simulink model "ortho_CAN_controlV2"  (R2016b)
settings: Solver=FixedStepDiscrete  StartTime=0.0  StopTime=180  FixedStep=.001  RelTol=1e-3  EnableMultiTasking=on
values from neighbouring files (symbols this model uses):
  rho1 = (rho01*(1-d(3)))+(rho11*d(3))    [fcn.m]
  rho2 = (rho02*(1-d(3)))+(rho12*d(3))    [fcn.m]
  theta1 = (theta01*(1-d(3)))+(theta11*d(3))    [fcn.m]
  theta2 = (theta02*(1-d(3)))+(theta12*d(3))    [fcn.m]
undefined symbols (not defined in the file or in its folder): bit, fdesignblkfcn, gcbh, rho_end, Standard, theta_end
libraries: slrtlib x7, simulink x6, slrtsoftinglib x3, xpcnilib x3, canmsglib x2
(part 1 of 2)
settings Model: xpc_rtwmakecfg_data=_xpccanac2pci_  SimulationMode=external  Creator=dholley  LastModifiedBy=1108gotthem
settings SolverCC: EnableConcurrentExecution=on  AlgebraicLoopSolver=LineSearch
settings DataIOCC: LimitDataPoints=on  SaveFormat=Array  SaveOutput=off  SignalLogging=off  DSMLogging=off
settings OptimizationCC: BlockReduction=off  OptimizeBlockIOStorage=off  BufferReuse=off  GlobalBufferReuse=off  ExpressionFolding=off  LocalBlockOutputs=off
settings DebuggingCC: UnderspecifiedInitializationDetection=Classic  MergeDetectMultiDrivingBlocksExec=none  SolverPrmCheckMsg=warning  StateNameClashWarn=warning  SFUnexpectedBacktrackingDiag=warning  SFNoUnconditionalDefaultTransitionDiag=warning  SFExecutionAtInitializationDiag=none
settings HardwareCC: ProdBitPerPointer=32  ProdBitPerSizeT=32  ProdBitPerPtrDiffT=32  ProdLargestAtomicFloat=None  ProdWordSize=32  ProdLongLongMode=on  ProdHWDeviceType=Generic->32-bit x86 compatible
settings ModelReferenceCC: PropagateSignalLabelsOutOfModel=off
settings RTWCC: SystemTargetFile=slrt.tlc  TemplateMakefile=slrt_default_tmf  Description=Simulink Real-Time  RTWCompilerOptimization=on
settings SimulinkRealTimeCC: RL32LogBufSizeModifier=6120000  xPCisModelTimeout=off  xPCModelTimeoutSecs=120
settings ConfigComp: CovMetricSettings=dw  CovHtmlReporting=on  CovSaveCumulativeToWorkspaceVar=on  CovSaveSingleToWorkspaceVar=on  CovExternalEMLEnable=off

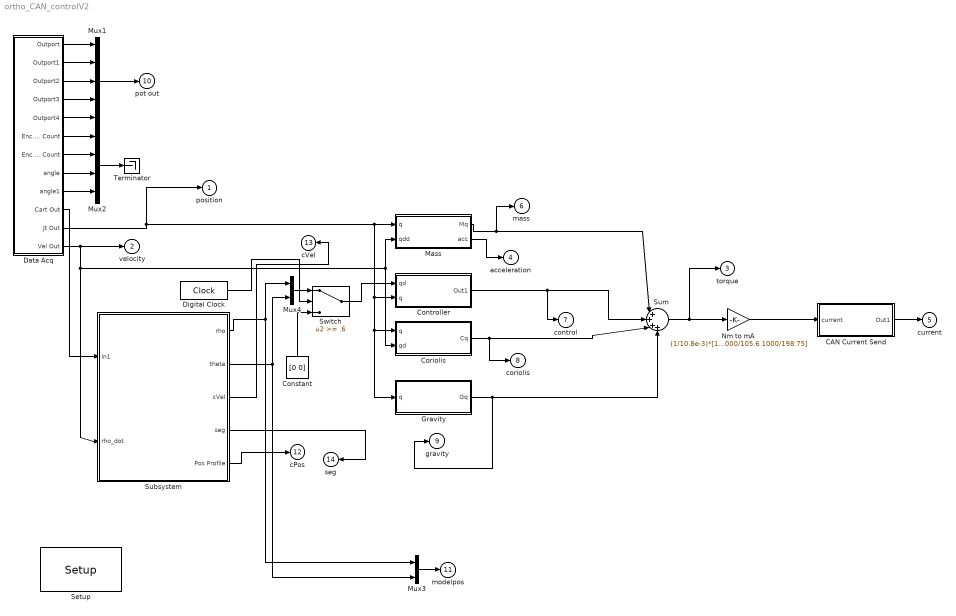
== system ortho_CAN_controlV2 ==
  CAN Current Send : Subsystem
  Constant : Constant  Value=[0 0]
  Controller : Subsystem  TreatAsAtomicUnit=on
      settings: RTWSystemCode=Inline
  Coriolis : Subsystem  TreatAsAtomicUnit=on
      settings: RTWSystemCode=Inline
  Data Acq : Subsystem
  Digital Clock : DigitalClock  SampleTime=.001
  Gravity : Subsystem  TreatAsAtomicUnit=on
      settings: RTWSystemCode=Inline
  Mass : Subsystem  TreatAsAtomicUnit=on
      settings: RTWSystemCode=Inline
  Mux1 : Mux  Inputs=5
  Mux2 : Mux
  Mux3 : Mux  Inputs=2
  Mux4 : Mux  Inputs=2
  Nm to mA : Gain  Gain=(1/10.8e-3)*[1000/105.6 1000/198.75]
  "Setup " : slrtsoftinglib/CAN-AC2-PCI SJA 1000/Setup   board=1  can1bus=Highspeed (ISO 11898)  can1Baudrate=1 MBaud  can1UserBR=[1,1,4,3]  can2bus=Highspeed (ISO 11898)  can2Baudrate=1 MBaud  can2UserBR=[1,1,4,3]  init=pdo_start  term=pdo_stop  bus_off_out=off  bus_off_rec=Off  ioBaseAddress=-1
  Subsystem : Subsystem
  Sum : Sum  Inputs=|++++
  Switch : Switch  Threshold=.6  SampleTime=.001
  Terminator : Terminator
  position : Outport  InitialOutput=0
  velocity : Outport  Port=2  InitialOutput=0
  torque : Outport  Port=3  InitialOutput=0
  acceleration : Outport  Port=4  InitialOutput=0
  current : Outport  Port=5  InitialOutput=0
  mass : Outport  Port=6  InitialOutput=0
  control : Outport  Port=7  InitialOutput=0
  coriolis : Outport  Port=8  InitialOutput=0
  gravity : Outport  Port=9  InitialOutput=0
  "pot out " : Outport  Port=10  InitialOutput=0
  "modelpos " : Outport  Port=11  InitialOutput=0
  cPos : Outport  Port=12  InitialOutput=0
  cVel : Outport  Port=13  InitialOutput=0
  "seg " : Outport  Port=14  InitialOutput=0
  wires:
  Gravity/1(Gq) -> Sum/4, gravity/1
  Coriolis/1(Cq) -> coriolis/1, Sum/3
  Mass/1(Mq) -> Sum/1, mass/1
  Mass/2(acc) -> acceleration/1
  CAN Current Send/1(Out1) -> current/1
  Data Acq/12(Vel Out) -> velocity/1, Subsystem/2(rho_dot), Coriolis/2(qd), Mass/2(qdd)
  Data Acq/11(Jt Out) -> position/1, Gravity/1(q), Coriolis/1(q), Controller/2(q), Mass/1(q)
  Data Acq/1(Outport) -> Mux1/1
  Data Acq/2(Outport1) -> Mux1/2
  Data Acq/3(Outport2) -> Mux1/3
  Data Acq/4(Outport3) -> Mux1/4
  Data Acq/5(Outport4) -> Mux1/5
  Mux1/1 -> "pot out "/1
  Data Acq/6(Enc. 1 Count) -> Mux2/1
  Data Acq/8(angle) -> Mux2/3
  Mux2/1 -> Terminator/1
  Controller/1(Out1) -> control/1, Sum/2
  Subsystem/1(rho) -> Mux4/1, Mux3/1
  Subsystem/2("theta ") -> Mux4/2, Mux3/2
  Mux3/1 -> "modelpos "/1
  Nm to mA/1 -> CAN Current Send/1(current)
  Sum/1 -> torque/1, Nm to mA/1
  Subsystem/3("cVel ") -> cVel/1
  Subsystem/4("seg ") -> "seg "/1
  Data Acq/7(Enc. 2 Count) -> Mux2/2
  Data Acq/9(angle1) -> Mux2/4
  Data Acq/10(Cart Out) -> Subsystem/1(In1)
  Subsystem/5(Pos Profile) -> cPos/1
  Mux4/1 -> Switch/1
  Switch/1 -> Controller/1(qd)
  Constant/1 -> Switch/3
  Digital Clock/1 -> Switch/2

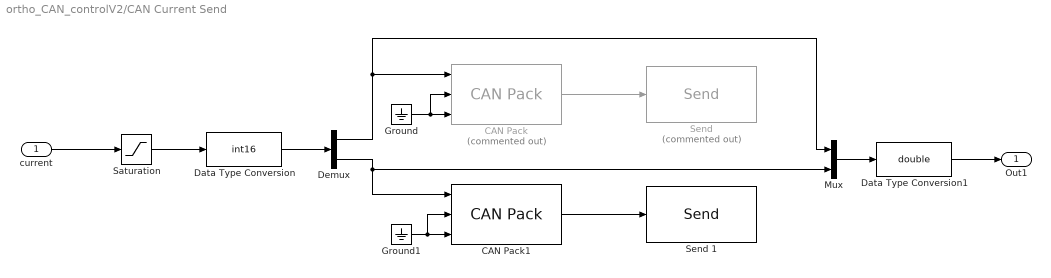
== system ortho_CAN_controlV2/CAN Current Send ==
  current : Inport
  CAN Pack : canmsglib/CAN Pack  Commented=on  MsgList=(none)  MsgName=CAN Msg  MsgIDType=Standard (11-bit identifier)  MsgIdentifier=hex2dec('202')  MsgLength=8  SignalInfo=current$0$16$1$1$1$0$1$0$-Inf$Inf$#null$16$32$1$1$1$0$1$0$-Inf$Inf$#null2$48$16$1$1$1$0$1$0$-Inf$Inf$#  NSignals=3  StartBits=str2num('[int32(0);int32(16);int32(48)]')  SignalSizes=str2num('[int32(16);int32(32);int32(16)]')  ByteOrders=str2num('[int32(1);int32(1);int32(1)]')  DataTypes=str2num('[int32(1);int32(1);int32(1)]')  MultiplexTypes=str2num('[int32(1);int32(1);int32(1)]')  MultiplexValues=str2num('[double(0);double(0);double(0)]')  Factors=str2num('[double(1);double(1);double(1)]')  Offsets=str2num('[double(0);double(0);double(0)]')  Minimums=str2num('[double(-Inf);double(-Inf);double(-Inf)]')  Maximums=str2num('[double(Inf);double(Inf);double(Inf)]')  Remote=off
      settings: DataFormat=manually specified signals
  CAN Pack1 : canmsglib/CAN Pack  MsgList=(none)  MsgName=CAN Msg  MsgIDType=Standard (11-bit identifier)  MsgIdentifier=hex2dec('201')  MsgLength=8  SignalInfo=current$0$16$1$1$1$0$1$0$-Inf$Inf$#null$16$32$1$1$1$0$1$0$-Inf$Inf$#null2$48$16$1$1$1$0$1$0$-Inf$Inf$#  NSignals=3  StartBits=str2num('[int32(0);int32(16);int32(48)]')  SignalSizes=str2num('[int32(16);int32(32);int32(16)]')  ByteOrders=str2num('[int32(1);int32(1);int32(1)]')  DataTypes=str2num('[int32(1);int32(1);int32(1)]')  MultiplexTypes=str2num('[int32(1);int32(1);int32(1)]')  MultiplexValues=str2num('[double(0);double(0);double(0)]')  Factors=str2num('[double(1);double(1);double(1)]')  Offsets=str2num('[double(0);double(0);double(0)]')  Minimums=str2num('[double(-Inf);double(-Inf);double(-Inf)]')  Maximums=str2num('[double(Inf);double(Inf);double(Inf)]')  Remote=off
      settings: DataFormat=manually specified signals
  Data Type Conversion : DataTypeConversion  OutDataTypeStr=int16
  Data Type Conversion1 : DataTypeConversion  OutDataTypeStr=double
  Demux : Demux  Outputs=2
  Ground : Ground
  Ground1 : Ground
  Mux : Mux  Inputs=2
  Saturation : Saturate  UpperLimit=1700  LowerLimit=-1700
  "Send " : slrtsoftinglib/CAN-AC2-PCI SJA 1000/Send   Commented=on  board=1  canPort=CAN 1  range=Standard (11-bit)  ids=hex2dec('202')  sizes=[8]  output=off  ts=0.001  ididx=[2]
  Send 1 : slrtsoftinglib/CAN-AC2-PCI SJA 1000/Send   board=1  canPort=CAN 1  range=Standard (11-bit)  ids=hex2dec('201')  sizes=[8]  output=off  ts=0.001  ididx=[1]
  Out1 : Outport
  wires:
  current/1 -> Saturation/1
  CAN Pack/1 -> "Send "/1
  CAN Pack1/1 -> Send 1/1
  Ground/1 -> CAN Pack/2, CAN Pack/3
  Ground1/1 -> CAN Pack1/2, CAN Pack1/3
  Demux/1 -> CAN Pack/1, Mux/1
  Demux/2 -> Mux/2, CAN Pack1/1
  Saturation/1 -> Data Type Conversion/1
  Data Type Conversion/1 -> Demux/1
  Data Type Conversion1/1 -> Out1/1
  Mux/1 -> Data Type Conversion1/1

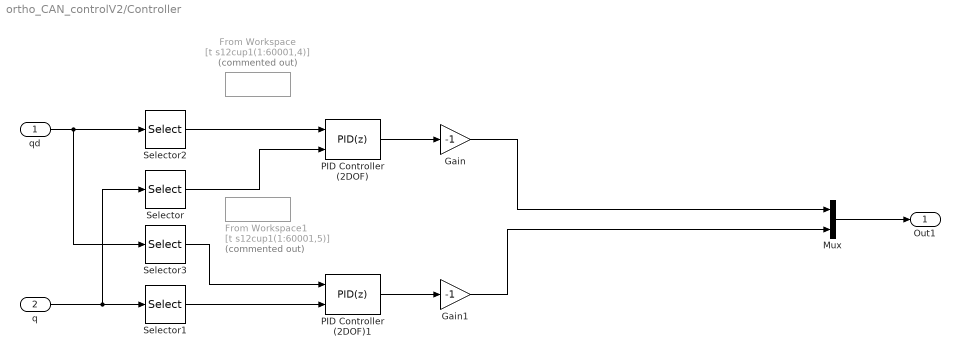
== system ortho_CAN_controlV2/Controller ==
  qd : Inport
  q : Inport  Port=2
  From Workspace : FromWorkspace  Commented=on  VariableName=[t s12cup1(1:60001,4)]  SampleTime=0
  From Workspace1 : FromWorkspace  Commented=on  VariableName=[t s12cup1(1:60001,5)]  SampleTime=0
  Gain : Gain  Gain=-1
  Gain1 : Gain  Gain=-1
  Mux : Mux  Inputs=2
  PID Controller (2DOF) : simulink/Continuous/PID Controller (2DOF)  Controller=PID  TimeDomain=Discrete-time  SampleTime=.001  IntegratorMethod=Forward Euler  FilterMethod=Forward Euler  Form=Parallel  UseFilter=on  ControllerParametersSource=internal  P=75  I=45  D=2  N=103  b=1  c=1  InitialConditionSource=internal  InitialConditionForIntegrator=0  InitialConditionForFilter=0  ExternalReset=none  LimitOutput=off  UpperSaturationLimit=inf  LowerSaturationLimit=-inf  LinearizeAsGain=on  AntiWindupMode=none  Kb=1  TrackingMode=off  Kt=1  PParamMin=[]  PParamMax=[]  IParamMin=[]  IParamMax=[]  DParamMin=[]  DParamMax=[]  NParamMin=[]  NParamMax=[]  bParamMin=[]  bParamMax=[]  cParamMin=[]  cParamMax=[]  KbParamMin=[]  KbParamMax=[]  KtParamMin=[]  KtParamMax=[]  POutMin=[]  POutMax=[]  IOutMin=[]  IOutMax=[]  DOutMin=[]  DOutMax=[]  NOutMin=[]  NOutMax=[]  bOutMin=[]  bOutMax=[]  cOutMin=[]  cOutMax=[]  KbOutMin=[]  KbOutMax=[]  KtOutMin=[]  KtOutMax=[]  IntegratorOutMin=[]  IntegratorOutMax=[]  FilterOutMin=[]  FilterOutMax=[]  SumOutMin=[]  SumOutMax=[]  Sum1OutMin=[]  Sum1OutMax=[]  Sum2OutMin=[]  Sum2OutMax=[]  Sum3OutMin=[]  Sum3OutMax=[]  SumI1OutMin=[]  SumI1OutMax=[]  SumI2OutMin=[]  SumI2OutMax=[]  SumI3OutMin=[]  SumI3OutMax=[]  SumDOutMin=[]  SumDOutMax=[]  SaturationOutMin=[]  SaturationOutMax=[]  IntegratorContinuousStateAttributes=''  IntegratorStateMustResolveToSignalObject=off  IntegratorRTWStateStorageClass=Auto  FilterContinuousStateAttributes=''  FilterStateMustResolveToSignalObject=off  FilterRTWStateStorageClass=Auto  DifferentiatorICPrevScaledInput=0  DifferentiatorOutMin=[]  DifferentiatorOutMax=[]
  PID Controller (2DOF)1 : simulink/Continuous/PID Controller (2DOF)  Controller=PID  TimeDomain=Discrete-time  SampleTime=.001  IntegratorMethod=Forward Euler  FilterMethod=Forward Euler  Form=Parallel  UseFilter=on  ControllerParametersSource=internal  P=30  I=20  D=3  N=100  b=1  c=1  InitialConditionSource=internal  InitialConditionForIntegrator=0  InitialConditionForFilter=0  ExternalReset=none  LimitOutput=off  UpperSaturationLimit=inf  LowerSaturationLimit=-inf  LinearizeAsGain=on  AntiWindupMode=none  Kb=1  TrackingMode=off  Kt=1  PParamMin=[]  PParamMax=[]  IParamMin=[]  IParamMax=[]  DParamMin=[]  DParamMax=[]  NParamMin=[]  NParamMax=[]  bParamMin=[]  bParamMax=[]  cParamMin=[]  cParamMax=[]  KbParamMin=[]  KbParamMax=[]  KtParamMin=[]  KtParamMax=[]  POutMin=[]  POutMax=[]  IOutMin=[]  IOutMax=[]  DOutMin=[]  DOutMax=[]  NOutMin=[]  NOutMax=[]  bOutMin=[]  bOutMax=[]  cOutMin=[]  cOutMax=[]  KbOutMin=[]  KbOutMax=[]  KtOutMin=[]  KtOutMax=[]  IntegratorOutMin=[]  IntegratorOutMax=[]  FilterOutMin=[]  FilterOutMax=[]  SumOutMin=[]  SumOutMax=[]  Sum1OutMin=[]  Sum1OutMax=[]  Sum2OutMin=[]  Sum2OutMax=[]  Sum3OutMin=[]  Sum3OutMax=[]  SumI1OutMin=[]  SumI1OutMax=[]  SumI2OutMin=[]  SumI2OutMax=[]  SumI3OutMin=[]  SumI3OutMax=[]  SumDOutMin=[]  SumDOutMax=[]  SaturationOutMin=[]  SaturationOutMax=[]  IntegratorContinuousStateAttributes=''  IntegratorStateMustResolveToSignalObject=off  IntegratorRTWStateStorageClass=Auto  FilterContinuousStateAttributes=''  FilterStateMustResolveToSignalObject=off  FilterRTWStateStorageClass=Auto  DifferentiatorICPrevScaledInput=0  DifferentiatorOutMin=[]  DifferentiatorOutMax=[]
  Selector : Selector  InputPortWidth=2  IndexOptions=Index vector (dialog)  Indices=[1]  OutputSizes=1
  Selector1 : Selector  InputPortWidth=2  IndexOptions=Index vector (dialog)  Indices=[2]  OutputSizes=1
  Selector2 : Selector  InputPortWidth=2  IndexOptions=Index vector (dialog)  Indices=[1]  OutputSizes=1
  Selector3 : Selector  InputPortWidth=2  IndexOptions=Index vector (dialog)  Indices=[2]  OutputSizes=1
  Out1 : Outport
  wires:
  q/1 -> Selector/1, Selector1/1
  Selector/1 -> PID Controller (2DOF)/2
  Mux/1 -> Out1/1
  Selector1/1 -> PID Controller (2DOF)1/2
  PID Controller (2DOF)/1 -> Gain/1
  PID Controller (2DOF)1/1 -> Gain1/1
  Gain/1 -> Mux/1
  Gain1/1 -> Mux/2
  qd/1 -> Selector3/1, Selector2/1
  Selector2/1 -> PID Controller (2DOF)/1
  Selector3/1 -> PID Controller (2DOF)1/1

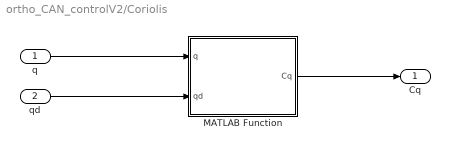
== system ortho_CAN_controlV2/Coriolis ==
  q : Inport
  qd : Inport  Port=2
  MATLAB Function : MATLAB Function  TreatAsAtomicUnit=on
  Cq : Outport
  wires:
  q/1 -> MATLAB Function/1(q)
  MATLAB Function/1(Cq) -> Cq/1
  qd/1 -> MATLAB Function/2(qd)

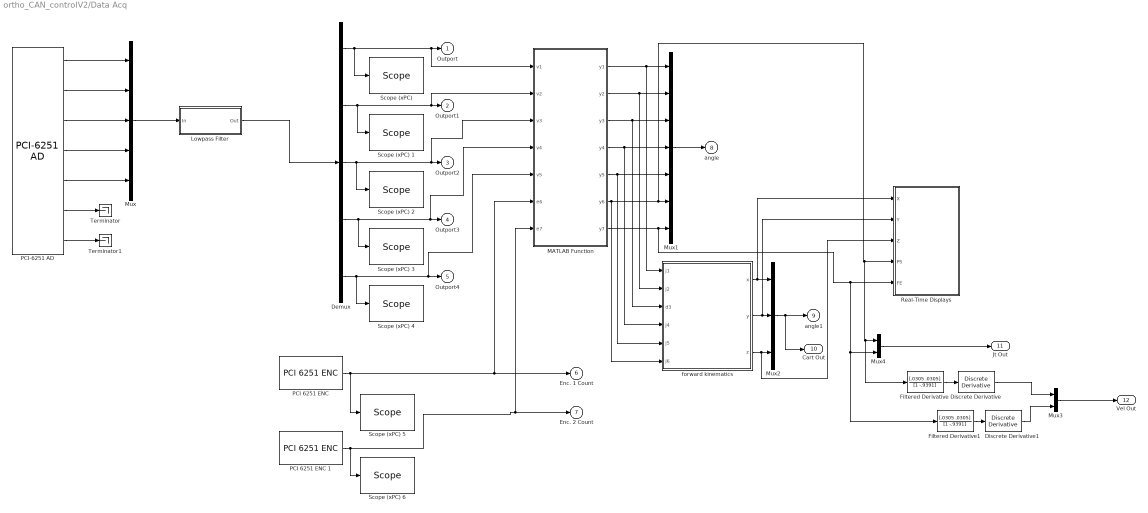
== system ortho_CAN_controlV2/Data Acq ==
  Demux : Demux  Outputs=5
  Discrete Derivative : simulink/Discrete/Discrete Derivative  gainval=1.0  ICPrevScaledInput=0.0  OutMin=[]  OutMax=[]  OutDataType=fixdt(1, 16)  OutScaling=2^-10  DoSatur=off
  Discrete Derivative1 : simulink/Discrete/Discrete Derivative  gainval=1.0  ICPrevScaledInput=0.0  OutMin=[]  OutMax=[]  OutDataType=fixdt(1, 16)  OutScaling=2^-10  DoSatur=off
  Filtered Derivative : DiscreteFilter  Numerator=[.0305 .0305]  Denominator=[1 -.9391]  SampleTime=0.001
  Filtered Derivative1 : DiscreteFilter  Numerator=[.0305 .0305]  Denominator=[1 -.9391]  SampleTime=0.001
  Lowpass Filter : Subsystem  DialogController=fdesignblkfcn  InitFcn=fdesignblkfcn(gcbh, {'InitFcn'});  mask(Lowpass Filter){}
      mask help: Design a lowpass filter
      settings: CopyFcn=fdesignblkfcn(gcbh, {'CopyFcn'});
      mask Help: helpview(mapfilelocation('dsp'), 'dsplowpassfilter');
      mask Display: disp('Lowpass')
  MATLAB Function : MATLAB Function  TreatAsAtomicUnit=on
  Mux : Mux  Inputs=5
  Mux1 : Mux  Inputs=7
  Mux2 : Mux  Inputs=3
  Mux3 : Mux  Inputs=2
  Mux4 : Mux  Inputs=2
  "PCI 6251 ENC " : xpcnilib/Incremental Encoder/PCI 6251 ENC   channel=1  countMode=Quadrature Mode x4  initCount=0  reload=off  indexPhase=A low B low  filter=None  sampleTime=0.001  slot=-1
  PCI 6251 ENC 1 : xpcnilib/Incremental Encoder/PCI 6251 ENC   channel=0  countMode=Quadrature Mode x4  initCount=0  reload=off  indexPhase=A low B low  filter=None  sampleTime=0.001  slot=-1
  PCI-6251 AD : xpcnilib/A//D/M Series/PCI-6251 AD  channel=[1,2,3,4,5,7,8]  range=[10,10,10,10,10,10,10]  coupling=[1,1,1,1,1,2,2]  scantime=5e-6  sampletime=0.001  slot=-1
  "Real-Time Displays " : Subsystem
  "Scope (xPC) " : slrtlib/Displays and Logging/Scope   scopeno=5  scopetype=Target  autostart=on  viewmode=Graphical rolling  formatstr='%15.6f'  grid=on  ylimits=[0,10]  nosamples=15001  noprepostsamples=0  interleave=1  triggermode=FreeRun  triggersignal=1  trigsignalfromport=off  triggerlevel=0.0  triggerslope=Either  triggerscope=1  triggersample=0  filename=data.dat  mode=Lazy  writesize=512  autorestart=off  dynamicfilemode=off  maxwritefilesize=512*1024^2
  Scope (xPC) 1 : slrtlib/Displays and Logging/Scope   scopeno=6  scopetype=Target  autostart=on  viewmode=Graphical rolling  formatstr='%15.6f'  grid=on  ylimits=[0,10]  nosamples=15001  noprepostsamples=0  interleave=1  triggermode=FreeRun  triggersignal=1  trigsignalfromport=off  triggerlevel=0.0  triggerslope=Either  triggerscope=1  triggersample=0  filename=data.dat  mode=Lazy  writesize=512  autorestart=off  dynamicfilemode=off  maxwritefilesize=512*1024^2
  Scope (xPC) 2 : slrtlib/Displays and Logging/Scope   scopeno=1  scopetype=Target  autostart=on  viewmode=Graphical rolling  formatstr='%15.6f'  grid=on  ylimits=[0,10]  nosamples=15001  noprepostsamples=0  interleave=1  triggermode=FreeRun  triggersignal=1  trigsignalfromport=off  triggerlevel=0.0  triggerslope=Either  triggerscope=1  triggersample=0  filename=data.dat  mode=Lazy  writesize=512  autorestart=off  dynamicfilemode=off  maxwritefilesize=512*1024^2
  Scope (xPC) 3 : slrtlib/Displays and Logging/Scope   scopeno=2  scopetype=Target  autostart=on  viewmode=Graphical rolling  formatstr='%15.6f'  grid=on  ylimits=[0,10]  nosamples=15001  noprepostsamples=0  interleave=1  triggermode=FreeRun  triggersignal=1  trigsignalfromport=off  triggerlevel=0.0  triggerslope=Either  triggerscope=1  triggersample=0  filename=data.dat  mode=Lazy  writesize=512  autorestart=off  dynamicfilemode=off  maxwritefilesize=512*1024^2
  Scope (xPC) 4 : slrtlib/Displays and Logging/Scope   scopeno=3  scopetype=Target  autostart=on  viewmode=Graphical rolling  formatstr='%15.6f'  grid=on  ylimits=[0,10]  nosamples=15001  noprepostsamples=0  interleave=1  triggermode=FreeRun  triggersignal=1  trigsignalfromport=off  triggerlevel=0.0  triggerslope=Either  triggerscope=1  triggersample=0  filename=data.dat  mode=Lazy  writesize=512  autorestart=off  dynamicfilemode=off  maxwritefilesize=512*1024^2
  Scope (xPC) 5 : slrtlib/Displays and Logging/Scope   scopeno=7  scopetype=Target  autostart=on  viewmode=Graphical rolling  formatstr='%15.6f'  grid=on  ylimits=[-15000,15000]  nosamples=15001  noprepostsamples=0  interleave=1  triggermode=FreeRun  triggersignal=1  trigsignalfromport=off  triggerlevel=0.0  triggerslope=Either  triggerscope=1  triggersample=0  filename=data.dat  mode=Lazy  writesize=512  autorestart=off  dynamicfilemode=off  maxwritefilesize=512*1024^2
  Scope (xPC) 6 : slrtlib/Displays and Logging/Scope   scopeno=4  scopetype=Target  autostart=on  viewmode=Graphical rolling  formatstr='%15.6f'  grid=on  ylimits=[-40000,40000]  nosamples=15001  noprepostsamples=0  interleave=1  triggermode=FreeRun  triggersignal=1  trigsignalfromport=off  triggerlevel=0.0  triggerslope=Either  triggerscope=1  triggersample=0  filename=data.dat  mode=Lazy  writesize=512  autorestart=off  dynamicfilemode=off  maxwritefilesize=512*1024^2
  Terminator : Terminator
  Terminator1 : Terminator
  forward kinematics : MATLAB Function  TreatAsAtomicUnit=on
  Outport : Outport  InitialOutput=0
  Outport1 : Outport  Port=2  InitialOutput=0
  Outport2 : Outport  Port=3  InitialOutput=0
  Outport3 : Outport  Port=4  InitialOutput=0
  Outport4 : Outport  Port=5  InitialOutput=0
  Enc. 1 Count : Outport  Port=6  InitialOutput=0
  Enc. 2 Count : Outport  Port=7  InitialOutput=0
  angle : Outport  Port=8  InitialOutput=0
  angle1 : Outport  Port=9  InitialOutput=0
  Cart Out : Outport  Port=10
  Jt Out : Outport  Port=11
  Vel Out : Outport  Port=12
  wires:
  PCI-6251 AD/1 -> Mux/1
  PCI-6251 AD/2 -> Mux/2
  PCI-6251 AD/3 -> Mux/3
  PCI-6251 AD/4 -> Mux/4
  Demux/1 -> "Scope (xPC) "/1, MATLAB Function/1(v1), Outport/1
  Lowpass Filter/1(Out) -> Demux/1
  MATLAB Function/1(y1) -> forward kinematics/1(j1), Mux1/1
  MATLAB Function/2(y2) -> forward kinematics/2(j2), Mux1/2
  MATLAB Function/3(y3) -> forward kinematics/3(d3), Mux1/3
  MATLAB Function/4(y4) -> forward kinematics/4(j4), Mux1/4
  MATLAB Function/5(y5) -> forward kinematics/5(j5), Mux1/5
  Mux1/1 -> angle/1
  MATLAB Function/6(y6) -> forward kinematics/6(j6), Filtered Derivative/1, Mux4/1, "Real-Time Displays "/4(PS), Mux1/6
  MATLAB Function/7(y7) -> Filtered Derivative1/1, Mux4/2, "Real-Time Displays "/5(FE), Mux1/7
  PCI-6251 AD/5 -> Mux/5
  Mux/1 -> Lowpass Filter/1(In)
  Demux/2 -> Scope (xPC) 1/1, MATLAB Function/2(v2), Outport1/1
  Demux/3 -> Scope (xPC) 2/1, MATLAB Function/3(v3), Outport2/1
  Demux/4 -> Scope (xPC) 3/1, MATLAB Function/4(v4), Outport3/1
  Demux/5 -> Scope (xPC) 4/1, Outport4/1, MATLAB Function/5(v5)
  forward kinematics/1(x) -> "Real-Time Displays "/1(X), Mux2/1
  forward kinematics/2(y) -> "Real-Time Displays "/2(Y), Mux2/2
  forward kinematics/3(z) -> "Real-Time Displays "/3(Z), Mux2/3
  Mux2/1 -> Cart Out/1, angle1/1
  Filtered Derivative1/1 -> Discrete Derivative1/1
  Filtered Derivative/1 -> Discrete Derivative/1
  Discrete Derivative/1 -> Mux3/1
  Discrete Derivative1/1 -> Mux3/2
  Mux3/1 -> Vel Out/1
  Mux4/1 -> Jt Out/1
  "PCI 6251 ENC "/1 -> Scope (xPC) 5/1, MATLAB Function/6(e6), Enc. 1 Count/1
  PCI 6251 ENC 1/1 -> MATLAB Function/7(e7), Enc. 2 Count/1, Scope (xPC) 6/1
  PCI-6251 AD/6 -> Terminator/1
  PCI-6251 AD/7 -> Terminator1/1

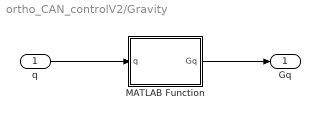
== system ortho_CAN_controlV2/Gravity ==
  q : Inport
  MATLAB Function : MATLAB Function  TreatAsAtomicUnit=on
  Gq : Outport
  wires:
  q/1 -> MATLAB Function/1(q)
  MATLAB Function/1(Gq) -> Gq/1

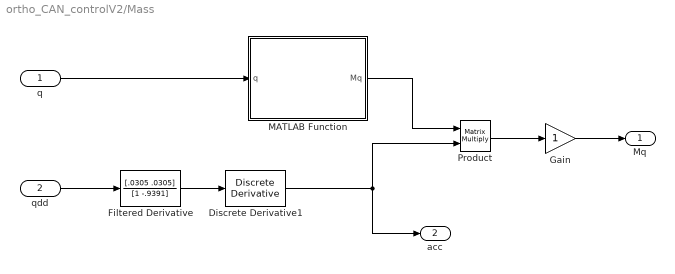
== system ortho_CAN_controlV2/Mass ==
  q : Inport
  qdd : Inport  Port=2
  Discrete Derivative1 : simulink/Discrete/Discrete Derivative  gainval=1.0  ICPrevScaledInput=0.0  OutMin=[]  OutMax=[]  OutDataType=fixdt(1, 16)  OutScaling=2^-10  DoSatur=off
  Filtered Derivative : DiscreteFilter  Numerator=[.0305 .0305]  Denominator=[1 -.9391]  SampleTime=0.001
  Gain : Gain
  MATLAB Function : MATLAB Function  TreatAsAtomicUnit=on
  Product : Product  Multiplication=Matrix(*)  RndMeth=Zero
  Mq : Outport
  acc : Outport  Port=2
  wires:
  q/1 -> MATLAB Function/1(q)
  MATLAB Function/1(Mq) -> Product/1
  Product/1 -> Gain/1
  Gain/1 -> Mq/1
  qdd/1 -> Filtered Derivative/1
  Discrete Derivative1/1 -> acc/1, Product/2
  Filtered Derivative/1 -> Discrete Derivative1/1

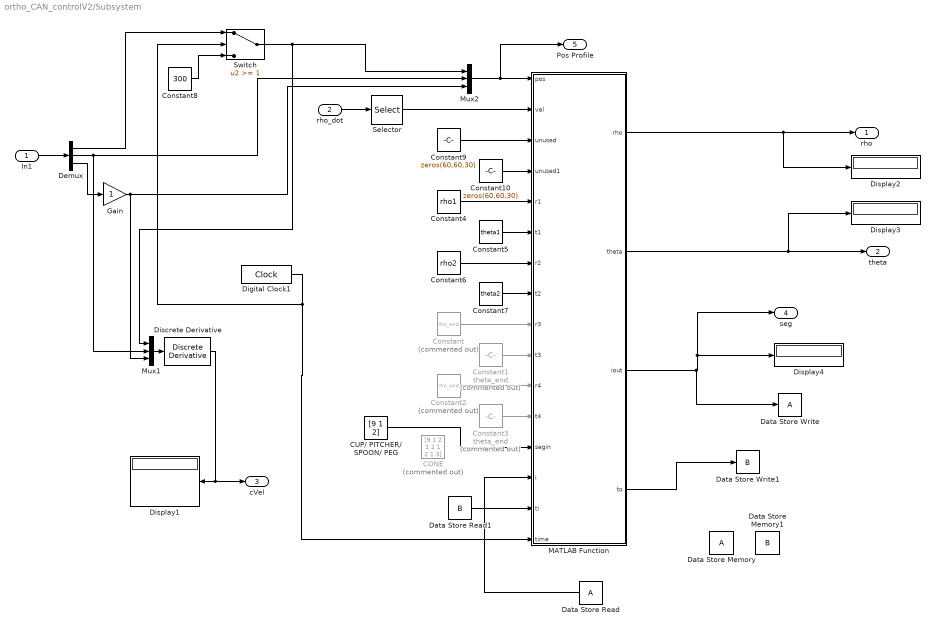
== system ortho_CAN_controlV2/Subsystem ==
  In1 : Inport
  rho_dot : Inport  Port=2
  "CONE " : Constant  Commented=on  Value=[9 1 2 1 2 1 2 1 3]  SampleTime=.001
  "CUP/ PITCHER/ SPOON/ PEG " : Constant  Value=[9 1 2]  SampleTime=.001
  Constant : Constant  Commented=on  Value=rho_end  VectorParams1D=off
  Constant1 : Constant  Commented=on  Value=theta_end  VectorParams1D=off
  Constant10 : Constant  Value=zeros(60,60,30)  VectorParams1D=off
  Constant2 : Constant  Commented=on  Value=rho_end  VectorParams1D=off
  Constant3 : Constant  Commented=on  Value=theta_end  VectorParams1D=off
  Constant4 : Constant  Value=rho1  VectorParams1D=off
  Constant5 : Constant  Value=theta1  VectorParams1D=off
  Constant6 : Constant  Value=rho2  VectorParams1D=off
  Constant7 : Constant  Value=theta2  VectorParams1D=off
  Constant8 : Constant  Value=300  SampleTime=.001
  Constant9 : Constant  Value=zeros(60,60,30)  VectorParams1D=off
  Data Store Memory : DataStoreMemory  ReadBeforeWriteMsg=warning  WriteAfterWriteMsg=warning  WriteAfterReadMsg=warning  InitialValue=1  ShowAdditionalParam=off
  Data Store Memory1 : DataStoreMemory  DataStoreName=B  ReadBeforeWriteMsg=warning  WriteAfterWriteMsg=warning  WriteAfterReadMsg=warning  InitialValue=-.4  ShowAdditionalParam=off
  Data Store Read : DataStoreRead  SampleTime=.001
  Data Store Read1 : DataStoreRead  DataStoreName=B  SampleTime=.001
  Data Store Write : DataStoreWrite  SampleTime=.001
  Data Store Write1 : DataStoreWrite  DataStoreName=B  SampleTime=.001
  Demux : Demux  Outputs=3
  Digital Clock1 : DigitalClock  SampleTime=.001
  Discrete Derivative : simulink/Discrete/Discrete Derivative  gainval=1.0  ICPrevScaledInput=0.0  InputProcessing=Inherited  OutMin=[]  OutMax=[]  OutDataType=fixdt(1, 16)  OutScaling=2^-10  DoSatur=off
  Display{1..4} (4 alike) : Display
  Gain : Gain  SampleTime=.001
  MATLAB Function : MATLAB Function  TreatAsAtomicUnit=on
  Mux1 : Mux  Inputs=3
  Mux2 : Mux  Inputs=3
  Selector : Selector  InputPortWidth=2  IndexOptions=Index vector (dialog)  Indices=1  OutputSizes=1
  Switch : Switch  Threshold=1  SampleTime=.001
  rho : Outport
  "theta " : Outport  Port=2
  "cVel " : Outport  Port=3
  "seg " : Outport  Port=4
  Pos Profile : Outport  Port=5
  wires:
  rho_dot/1 -> Selector/1
  Digital Clock1/1 -> Switch/2, MATLAB Function/16(time)
  Constant8/1 -> Switch/3
  Mux1/1 -> Discrete Derivative/1
  Constant9/1 -> MATLAB Function/3(unused)
  Constant10/1 -> MATLAB Function/4(unused1)
  Constant4/1 -> MATLAB Function/5(r1)
  Constant5/1 -> MATLAB Function/6(t1)
  Constant6/1 -> MATLAB Function/7(r2)
  MATLAB Function/3(iout) -> Data Store Write/1, "seg "/1, Display4/1
  MATLAB Function/4(to) -> Data Store Write1/1
  MATLAB Function/1(rho) -> Display2/1, rho/1
  MATLAB Function/2(theta) -> Display3/1, "theta "/1
  Constant7/1 -> MATLAB Function/8(t2)
  Constant3/1 -> MATLAB Function/12(t4)
  Constant2/1 -> MATLAB Function/11(r4)
  Constant1/1 -> MATLAB Function/10(t3)
  Constant/1 -> MATLAB Function/9(r3)
  Demux/1 -> Switch/1
  Demux/3 -> Gain/1
  Mux2/1 -> Pos Profile/1, MATLAB Function/1(pos)
  Switch/1 -> Mux1/1, Mux2/1
  Demux/2 -> Mux1/2, Mux2/2
  Gain/1 -> Mux1/3, Mux2/3
  Data Store Read1/1 -> MATLAB Function/15(ti)
  Data Store Read/1 -> MATLAB Function/14(i)
  Discrete Derivative/1 -> "cVel "/1, Display1/1
  In1/1 -> Demux/1
  "CUP/ PITCHER/ SPOON/ PEG "/1 -> MATLAB Function/13(segin)
  Selector/1 -> MATLAB Function/2(vel)

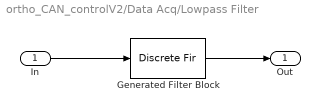
== system ortho_CAN_controlV2/Data Acq/Lowpass Filter ==
  In : Inport
  Generated Filter Block : DiscreteFir  Tag=BlockMethodSubSystem  Coefficients=[-0.00052324228244352597 -5.6057008840111622e-05 -5.9029960060090123e-05 -6.2089092415703651e-05 -6.5235172106602808e-05 -6.8468792239146433e-05 -7.1791170876184978e-05 -7.5199394031231657e-05 -7.8693485466635764e-05 -8.2278777605507031e-05 -8.595347305185517e-05 -8.9721309412065051e-05 -9.3578658035005043e-05 -9.7527959693077641e-05 -0.00010156823183841502 -0.00010570306844346472 -0.0001099328592674625 -0.00011425592773425428 -0.00011867203248127299 -0.0001231799968737532 -0.00012778728307383345 -0.00013249067611977418 -0.00013729314500949554 -0.00014218232070427767 -0.00014716926331734948 -0.00015225602378782298 -0.00015743218992457042 -0.00016269728987213943 -0.00016806238974750827 -0.00017352033232048865 -0.0001790541571821037 -0.00018469470695856038 -0.00019040984292100611 -0.00019621615780973255 -0.00020210453549572777 -0.00020807769136475324 -0.00021413162898923835 -0.00022026741549891577 -0.00022648545623399775 -0.00023278305632693007 -0.00023916116470940019 -0.00024561752902621861 -0.00025215563189431487 -0.00025877239732060919 -0.00026546870783869639 -0.00027224140486980879 -0.00027909126326666029 -0.00028601702953346975 -0.00029301423418495693 -0.0003000833632016655 -0.00030721562663037119 -0.00031442057334346384 -0.00032166470362155413 -0.0003289859106662829 -0.00033634358815721359 -0.00034374313095350431 -0.00035119427093453651 -0.00035868375459999696 -0.0003662039702031097 -0.00037376552352817309 -0.0003813735840803234 -0.00038901495643876518 -0.00039669544877577199 -0.00040441363753715757 -0.00041217530568567532 -0.00041997236920575794 -0.00042779681226945903 -0.00043563648316667354 -0.00044348025734073965 -0.00045131682050124572 -0.00045913146718169523 -0.00046691658695320793 -0.00047466786789203153 -0.00048240036364918733 -0.00049013557695491749 -0.00049790927995173621 -0.00050574222671454687 -0.00051362605492419008 -0.00052149568150616993 -0.00052920115935022743 -0.00053654954320442034 -0.00054357771054403859 -0.00055214790105943346 -0.00055916535223403136 -0.00056666427607138812 -0.00057404465564137052 -0.00058135307459826859 -0.00058858746107408311 -0.00059574654644921473 -0.00060282347017059977 -0.00060981028743565169 -0.00061670493558216505 -0.00062349928924097396 -0.000630192055063267 -0.00063677471765257723 -0.00064324342516180089 -0.00064958972288984044 -0.00065581029697547931 -0.0006619013208642088 -0.00066785686227762093 -0.00067367026968544099 -0.00067932944837409447 -0.00068483347458354069 -0.00069017350542580796 -0.00069535230042428028 -0.00070034879032750846 -0.00070516462522351693 -0.00070979980509052972 -0.00071424020173444002 -0.00071847608015420902 -0.00072251270665083943 -0.00072634337800568096 -0.00072994321245200037 -0.00073333574344273337 -0.00073649156348525686 -0.00073941703893840895 -0.00074210053887124113 -0.00074453916177031048 -0.00074672281031526401 -0.00074864519360783878 -0.00075030132489939145 -0.00075168278519708134 -0.00075278399298329122 -0.00075359502155582811 -0.00075411336084044384 -0.00075433142515719212 -0.00075424619678480674 -0.00075384983500808959 -0.00075313851527801946 -0.0007521083156189119 -0.0007507511200035438 -0.00074906499149087695 -0.00074703433019716707 -0.00074467569886822607 -0.00074193430250794738 -0.00073886247530116969 -0.00073541239059260954 -0.00073157897963701992 -0.0007273769919590344 -0.00072279421000670443 -0.00071781259232127099 -0.00071243669254971711 -0.00070667704483942564 -0.00070052009746154594 -0.00069396076402879247 -0.00068698617116579529 -0.00067959495504656586 -0.00067177723621101009 -0.00066352416222824231 -0.0006548251523169538 -0.00064567650220373897 -0.00063608395400448962 -0.00062605373231083893 -0.00061559312159697338 -0.00060469234669886644 -0.00059333532482305806 -0.00058149012821433687 -0.00056914033755682623 -0.00055628848147566494 -0.00054297275957292416 -0.00052924873470221775 -0.00051510617355876131 -0.0005003889172763155 -0.00048493969539900724 -0.00046944146128394216 -0.00045313869696779349 -0.0004364405176052949 ...(+12253 chars)]
  Out : Outport
  wires:
  In/1 -> Generated Filter Block/1
  Generated Filter Block/1 -> Out/1

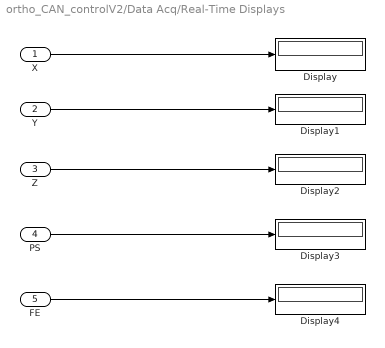
== system ortho_CAN_controlV2/Data Acq/Real-Time Displays  ==
  X : Inport
  Y : Inport  Port=2
  Z : Inport  Port=3
  PS : Inport  Port=4
  FE : Inport  Port=5
  Display{,1..4} (5 alike) : Display
  wires:
  Y/1 -> Display1/1
  Z/1 -> Display2/1
  PS/1 -> Display3/1
  FE/1 -> Display4/1
  X/1 -> Display/1

== matlab function ortho_CAN_controlV2/Coriolis/MATLAB Function ==
  data: q input; Cq output; qd input
function Cq = Coriolis(q,qd)
%#codegen

weight=(72.57);%kg
hand_length=(.175);%m
hand_width=(.082);%m

s7=sin(q(2));
c7=cos(q(2));
a7cm=-.00458;
d7cm=-.00285;
a6=.03952;
m7=.2256; %kg

hand_xcom=0;
hand_ycom=-hand_length*.468;
hand_zcom=hand_width/2;
hand_mass=weight*.00575;

com7=[a7cm;-.03363;d7cm]*m7 + [hand_xcom;hand_ycom;hand_zcom]*hand_mass/(m7 + hand_mass);

%Centrifugal
c112=-m7*com7(1)^2*s7*c7;
C1C2=[0 0;c112 0];

%Coriolis
c121=-m7*com7(1)^2*s7*c7;
c122=m7*com7(1)*com7(3)*c7;
C22=[c121;c122];

Cq=C22*(qd(1)*qd(2)) + C1C2*[qd(1)^2;qd(2)^2];

== matlab function ortho_CAN_controlV2/Mass/MATLAB Function ==
  data: q input; Mq output
function Mq  = massmatrix(q)

%%Input Metrics
height=(1.6764);%m
weight=(72.57);%kg
hand_length=(.175);%m
hand_width=(.082);%m
hand_thick=(.028);%m

% s1=sind(q(1));
% c1=cosd(q(1));
% s2=sind(q(2));
% c2=cosd(q(2));
% s4=sind(q(4));
% c4=cosd(q(4));
% s5=sind(q(5));
% c5=cosd(q(5));
s6=sin(q(1));
c6=cos(q(1));
s7=sin(q(2));
c7=cos(q(2));

m6=.4242; %kg
m7=.2256; %kg

%in m
a6cm=.02382;
d6cm=.04397;
a7cm=-.00458;
d7cm=-.00285;
d6=.06708;
a6=.03952;
a5=.12051;
d4=.04586;
a2=.37546;
d1=.33655;

%Forearm Inertia
forearm_length=height*.1585;
forearm_mass=weight*.016;
forearm_volume=forearm_mass/1062;
forearm_radius=sqrt(forearm_volume/(pi*forearm_length));

arm_zcom=d6-(forearm_length*.568);
arm_xcom=a6-forearm_radius;
arm_ycom=0;


kx_forearm=forearm_radius*.276;
ky_forearm=forearm_radius*.265;
kz_forearm=forearm_length*.121;
Ixx_forearm=forearm_mass*kx_forearm^2 + forearm_mass*arm_zcom^2;
Iyy_forearm=forearm_mass*ky_forearm^2 + forearm_mass*(arm_xcom^2 + arm_zcom^2);
Izz_forearm=forearm_mass*kz_forearm^2 + forearm_mass*arm_xcom^2;
Ixy_forearm=0;
Ixz_forearm=forearm_mass*arm_xcom*arm_zcom;
Iyz_forearm=0;

I_forearm=[Ixx_forearm,-Ixy_forearm,-Ixz_forearm;-Ixy_forearm,Iyy_forearm,-Iyz_forearm;-Ixz_forearm,-Iyz_forearm,Izz_forearm];

%Hand Inertia
hand_xcom=0;
hand_ycom=-hand_length*.468;
hand_zcom=hand_width/2;
hand_mass=weight*.00575;

kx_hand=hand_thick*.235;
ky_hand=hand_length*.184;
kz_hand=hand_width*.288;
Ixx_hand=hand_mass*kx_hand^2 + hand_mass*(hand_ycom^2 + hand_zcom^2);
Iyy_hand=hand_mass*ky_hand^2 + hand_mass*hand_zcom^2;
Izz_hand=hand_mass*kz_hand^2 + hand_mass*hand_ycom^2;
Ixy_hand=0;
Ixz_hand=0;
Iyz_hand=hand_mass*hand_ycom*hand_zcom;

I_hand=[Ixx_hand,-Ixy_hand,-Ixz_hand;-Ixy_hand,Iyy_hand,-Iyz_hand;-Ixz_hand,-Iyz_hand,Izz_hand];


I6=[2.259e-3 -7.049e-5 -9.252e-5;-7.049e-5 2.091e-3 -4.603e-4;-9.252e-5 -4.603e-4 8.911e-4];
I7=[7.022e-4 8.207e-5 -2.535e-5;8.207e-5 1.675e-4 -1.046e-4;-2.535e-5 -1.046e-4 6.273e-4];

%Forward Kinematics for Positioning
% x=-a5*c1*s2*c5 - a5*s5*(s1*c4 - c1*c2*s4) - d4*c1*s2 + d3*c1*c2 + a2*c1*c2;
% y=-a5*s1*s2*c5 + a5*s5*(c1*c4 + s1*c2*c4) - d4*s1*s2 + d3*s1*c2 + a2*s1*c2;
% z=-a5*c2*c5 - a5*s2*s4*s5 - d4*c2 - d3*s2 - a2*s2 + d1;

%Modified Center of Mass Location
com6=[a6cm;-.01547;d6cm]*m6 + [arm_xcom;arm_ycom;arm_zcom]*forearm_mass/(m6 + forearm_mass);
com7=[a7cm;-.03363;d7cm]*m7 + [hand_xcom;hand_ycom;hand_zcom]*hand_mass/(m7 + hand_mass);

%Jacobian
Jv1=[-com6(1)*s6,0;com6(1)*c6,0;0,0];
Jv2=[-com7(1)*c6*c7 + com7(3)*s6 - a6*c6,com7(1)*s6*s7;-com7(1)*s6*c7 - com7(3)*c6 - a6*s6,-com7(1)*c6*s7;0,-com7(1)*c7];

Jw1=[0,0;0,0;1,0];
Jw2=[0,-c6;0,-s6;1,0];

%Rotation Matrix
R6=[-s6,0,-c6;c6,0,-s6;0,-1,0];

D6=m6*(Jv1'*Jv1)+Jw1'*(I6 + I_forearm)*Jw1;
D7=m7*(Jv2'*Jv2)+Jw2'*R6*(I7 + I_hand)*R6'*Jw2;
D=D6+D7;%Mass Matrix

Mq=D;

== matlab function ortho_CAN_controlV2/Gravity/MATLAB Function ==
  data: q input; Gq output
function Gq = Gravity(q)
%#codegen

height=(1.6764);%m
weight=(72.57);%kg
hand_length=(.175);%m
hand_width=(.082);%m

s6=sin(q(1));
c6=cos(q(1));
s7=sin(q(2));
c7=cos(q(2));

m6=.4242; %kg
m7=.2256; %kg

a7cm=-.00458;
d7cm=-.00285;
a6=.03952;
d6=.06708;
a6cm=.01425;
d6cm=.04397;

forearm_length=height*.1585;
forearm_mass=weight*.016;
forearm_volume=forearm_mass/1062;
forearm_radius=sqrt(forearm_volume/(pi*forearm_length));
arm_zcom=d6-(forearm_length*.568);
arm_xcom=a6-forearm_radius;
arm_ycom=0;

hand_xcom=0;
hand_ycom=-hand_length*.468;
hand_zcom=hand_width/2;
hand_mass=weight*.00575;

com6=[a6cm;-.01547;d6cm]*m6 + [arm_xcom;arm_ycom;arm_zcom]*forearm_mass/(m6 + forearm_mass);
com7=[a7cm;-.03363;d7cm]*m7 + [hand_xcom;hand_ycom;hand_zcom]*hand_mass/(m7 + hand_mass);

%Jacobian
Jv1=[-com6(1)*s6,0;com6(1)*c6,0;0,0];
Jv2=[-com7(1)*c6*c7 + com7(3)*s6 - a6*s6,com7(1)*s6*s7;-com7(1)*s6*c7 - com7(3)*c6 + a6*c6,-com7(1)*c6*s7;0,-com7(1)*c7];

Gq=-((Jv1'*m6*[9.81;0;0]) + (Jv2'*m7*[0;0;-9.81]));

== matlab function ortho_CAN_controlV2/Data Acq/MATLAB Function ==
  data: v1 input; y1 output; v2 input; v3 input; v4 input; v5 input; y2 output; y3 output; y4 output; y5 output; e6 input; e7 input; y6 output; y7 output
function [y1,y2,y3,y4,y5,y6,y7] = volt2deg(v1,v2,v3,v4,v5,e6,e7)
%#codegen

%Enter Calibration Voltages
joint1_zero=7.3609;
joint1_25=8.0502;
joint2=4.353;
joint3_extended=6.6944;
joint3_retracted=0.36547;
joint4=8.8793;
joint5=5.6408;
%-----------------------------------------------
slope1245=(joint1_25 - joint1_zero)/25;
%slope3=(joint3_extended - joint3_retracted)/438; %original
slope3=(joint3_extended - joint3_retracted)/436.56; %new travel

joint1_os=joint1_zero;
%joint2_os=joint2 + (slope1245 * 5.6932); %original
joint2_os=joint2 + (slope1245 * 3.8); %new angle
joint4_os=joint4;
joint5_os=joint5;

y1=(joint1_os - v1)./slope1245;
y2=(joint2_os - v2)./slope1245;
y3=(v3 - 1.9473)./slope3;
y4=(v4 - joint4_os)./slope1245;
y5=(v5 - joint5_os)./slope1245;
y6=(pi/180)*(30/18750).*e6;
y7=(pi/180)*(30/33920).*e7;
